simulink model "lab6"  (R2021b)
settings: Solver=ode4  StartTime=0.0  StopTime=400  FixedStep=0.01  RelTol=1e-3
model workspace (MAT data in the model file):
  Ti = 200
values from neighbouring files (symbols this model uses):
  ddMax = 3    [sysdata.m]
  deltaMax = 30    [sysdata.m]
  fConst = 0    [sysdata.m]
  K = 0.08    [sysdata.m]
  Kaw = 1    [lab6go.m]
  Kc = 0.7045    [sysdata.m]
  phiZad = 30    [sysdata.m]
  Toc = 5    [sysdata.m]
  Tr = 1    [sysdata.m]
  Ts = 18    [sysdata.m]
settings Model: Creator=valeria  LastModifiedBy=Ivan
settings SolverCC: AlgebraicLoopSolver=TrustRegion
settings DebuggingCC: SFMachineParentedDataDiag=warning

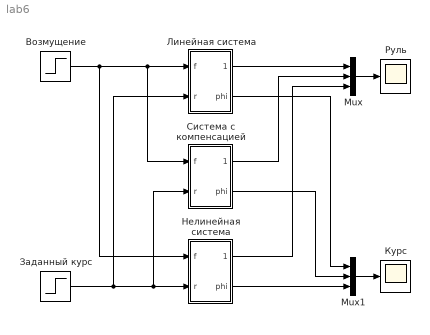
== system lab6 ==
  Mux : Mux  Inputs=3
  Mux1 : Mux  Inputs=3
  Возмущение : Step  Time=0  After=fConst  SampleTime=0
  Заданный курс : Step  Time=0  After=phiZad  SampleTime=0
  Курс : Scope
  Линейная система : Subsystem
  Нелинейная система : Subsystem
  Руль : Scope
  Система с компенсацией : Subsystem
  wires:
  Возмущение/1 -> Система с компенсацией/1(f), Линейная система/1(f), Нелинейная система/1(f)
  Mux/1 -> Руль/1
  Mux1/1 -> Курс/1
  Линейная система/1(delta) -> Mux/1
  Система с компенсацией/1(delta) -> Mux/2
  Нелинейная система/1(delta) -> Mux/3
  Нелинейная система/2(phi) -> Mux1/3
  Система с компенсацией/2(phi) -> Mux1/2
  Линейная система/2(phi) -> Mux1/1
  Заданный курс/1 -> Линейная система/2(r), Система с компенсацией/2(r), Нелинейная система/2(r)

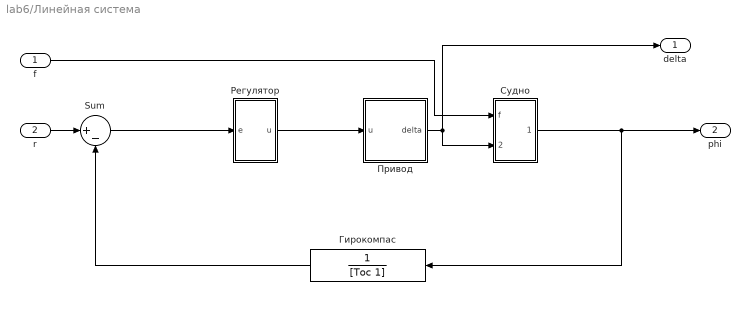
== system lab6/Линейная система ==
  f : Inport
  r : Inport  Port=2
  " Гирокомпас" : TransferFcn  Denominator=[Toc 1]
  Sum : Sum  Inputs=|+-
  Привод : Subsystem
  Регулятор : Subsystem
  Судно : Subsystem
  delta : Outport
  phi : Outport  Port=2
  wires:
  r/1 -> Sum/1
  Судно/1(phi) -> phi/1, " Гирокомпас"/1
  " Гирокомпас"/1 -> Sum/2
  Привод/1(delta) -> delta/1, Судно/2(delta)
  f/1 -> Судно/1(f)
  Sum/1 -> Регулятор/1(e)
  Регулятор/1(u) -> Привод/1(u)

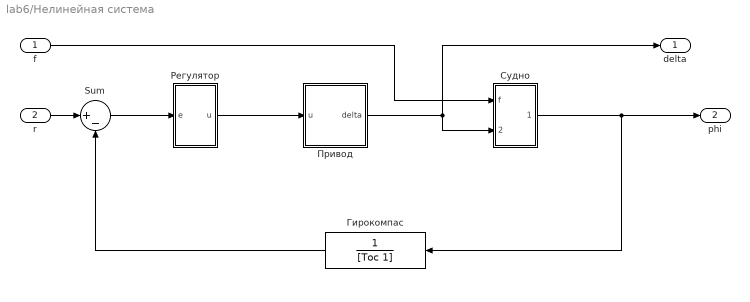
== system lab6/Нелинейная система ==
  f : Inport
  r : Inport  Port=2
  " Гирокомпас" : TransferFcn  Denominator=[Toc 1]
  Sum : Sum  Inputs=|+-
  Привод : Subsystem
  Регулятор : Subsystem
  Судно : Subsystem
  delta : Outport
  phi : Outport  Port=2
  wires:
  r/1 -> Sum/1
  Судно/1(phi) -> phi/1, " Гирокомпас"/1
  " Гирокомпас"/1 -> Sum/2
  Привод/1(delta) -> delta/1, Судно/2(delta)
  f/1 -> Судно/1(f)
  Sum/1 -> Регулятор/1(e)
  Регулятор/1(u) -> Привод/1(u)

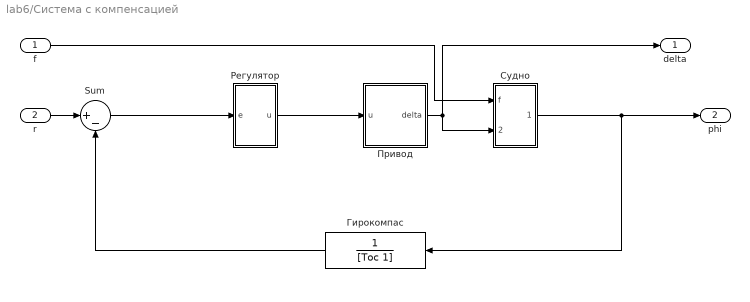
== system lab6/Система с компенсацией ==
  f : Inport
  r : Inport  Port=2
  " Гирокомпас" : TransferFcn  Denominator=[Toc 1]
  Sum : Sum  Inputs=|+-
  Привод : Subsystem
  Регулятор : Subsystem
  Судно : Subsystem
  delta : Outport
  phi : Outport  Port=2
  wires:
  r/1 -> Sum/1
  Судно/1(phi) -> phi/1, " Гирокомпас"/1
  " Гирокомпас"/1 -> Sum/2
  Привод/1(delta) -> delta/1, Судно/2(delta)
  f/1 -> Судно/1(f)
  Sum/1 -> Регулятор/1(e)
  Регулятор/1(u) -> Привод/1(u)

== system lab6/Линейная система/Привод ==
  u : Inport
  Привод : TransferFcn  Denominator=[Tr 1]
  delta : Outport
  wires:
  Привод/1 -> delta/1
  u/1 -> Привод/1

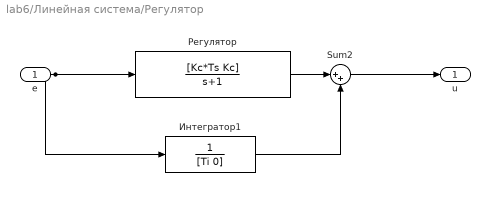
== system lab6/Линейная система/Регулятор ==
  e : Inport
  " Интегратор1" : TransferFcn  Denominator=[Ti 0]
  Sum2 : Sum  Inputs=|++
  Регулятор : TransferFcn  Numerator=[Kc*Ts Kc]  Denominator=[1 1]
  u : Outport
  wires:
  " Интегратор1"/1 -> Sum2/2
  e/1 -> " Интегратор1"/1, Регулятор/1
  Регулятор/1 -> Sum2/1
  Sum2/1 -> u/1

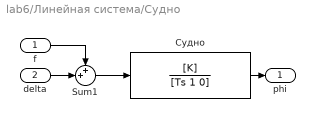
== system lab6/Линейная система/Судно ==
  f : Inport
  delta : Inport  Port=2
  Sum1 : Sum  Inputs=++|
  Судно : TransferFcn  Numerator=[K]  Denominator=[Ts 1 0]
  phi : Outport
  wires:
  Sum1/1 -> Судно/1
  Судно/1 -> phi/1
  delta/1 -> Sum1/2
  f/1 -> Sum1/1

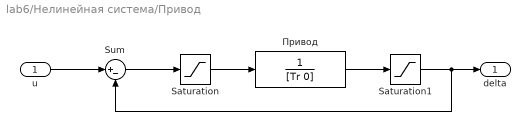
== system lab6/Нелинейная система/Привод ==
  u : Inport
  Saturation : Saturate  UpperLimit=+ddMax  LowerLimit=-ddMax
  Saturation1 : Saturate  UpperLimit=+deltaMax  LowerLimit=-deltaMax
  Sum : Sum  Inputs=|+-
  Привод : TransferFcn  Denominator=[Tr 0]
  delta : Outport
  wires:
  u/1 -> Sum/1
  Sum/1 -> Saturation/1
  Saturation/1 -> Привод/1
  Привод/1 -> Saturation1/1
  Saturation1/1 -> Sum/2, delta/1

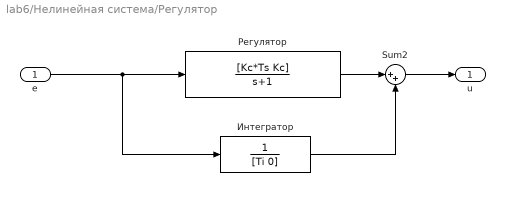
== system lab6/Нелинейная система/Регулятор ==
  e : Inport
  " Интегратор" : TransferFcn  Denominator=[Ti 0]
  Sum2 : Sum  Inputs=|++
  Регулятор : TransferFcn  Numerator=[Kc*Ts Kc]  Denominator=[1 1]
  u : Outport
  wires:
  " Интегратор"/1 -> Sum2/2
  e/1 -> Регулятор/1, " Интегратор"/1
  Регулятор/1 -> Sum2/1
  Sum2/1 -> u/1

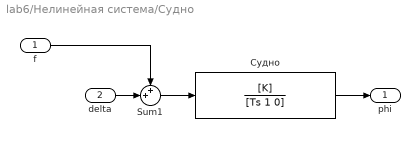
== system lab6/Нелинейная система/Судно ==
  f : Inport
  delta : Inport  Port=2
  Sum1 : Sum  Inputs=++|
  Судно : TransferFcn  Numerator=[K]  Denominator=[Ts 1 0]
  phi : Outport
  wires:
  Sum1/1 -> Судно/1
  Судно/1 -> phi/1
  delta/1 -> Sum1/2
  f/1 -> Sum1/1

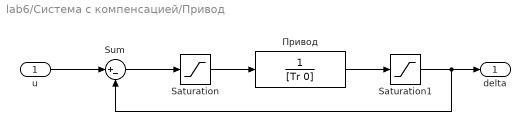
== system lab6/Система с компенсацией/Привод ==
  u : Inport
  Saturation : Saturate  UpperLimit=+ddMax  LowerLimit=-ddMax
  Saturation1 : Saturate  UpperLimit=+deltaMax  LowerLimit=-deltaMax
  Sum : Sum  Inputs=|+-
  Привод : TransferFcn  Denominator=[Tr 0]
  delta : Outport
  wires:
  u/1 -> Sum/1
  Sum/1 -> Saturation/1
  Saturation/1 -> Привод/1
  Привод/1 -> Saturation1/1
  Saturation1/1 -> Sum/2, delta/1

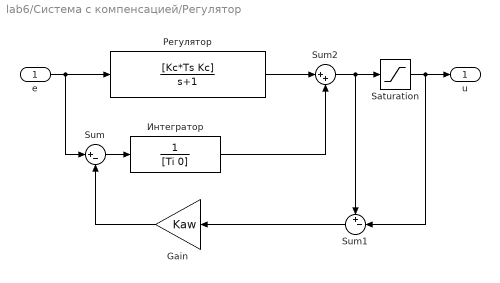
== system lab6/Система с компенсацией/Регулятор ==
  e : Inport
  " Интегратор" : TransferFcn  Denominator=[Ti 0]
  Gain : Gain  Gain=Kaw
  Saturation : Saturate  UpperLimit=30  LowerLimit=-30
  Sum : Sum  Inputs=|+-
  Sum1 : Sum  Inputs=+-|
  Sum2 : Sum  Inputs=|++
  Регулятор : TransferFcn  Numerator=[Kc*Ts Kc]  Denominator=[1 1]
  u : Outport
  wires:
  " Интегратор"/1 -> Sum2/2
  e/1 -> Регулятор/1, Sum/1
  Регулятор/1 -> Sum2/1
  Sum2/1 -> Saturation/1, Sum1/1
  Sum/1 -> " Интегратор"/1
  Saturation/1 -> Sum1/2, u/1
  Sum1/1 -> Gain/1
  Gain/1 -> Sum/2

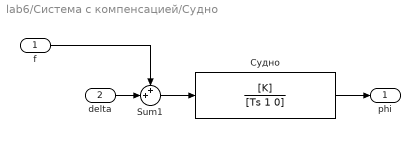
== system lab6/Система с компенсацией/Судно ==
  f : Inport
  delta : Inport  Port=2
  Sum1 : Sum  Inputs=++|
  Судно : TransferFcn  Numerator=[K]  Denominator=[Ts 1 0]
  phi : Outport
  wires:
  Sum1/1 -> Судно/1
  Судно/1 -> phi/1
  delta/1 -> Sum1/2
  f/1 -> Sum1/1
